simulink model "Set_arm_angles"  (R2020a)
settings: Solver=FixedStepAuto  StartTime=0.0  StopTime=30  FixedStep=0.5  RelTol=1e-3  EnableMultiTasking=on
values from neighbouring files (symbols this model uses):
  initial_elbow_angle = 0*pi/180    (= 0)    [Run_Initializer.m]
  initial_shoulder_angle = 0*pi/180    (= 0)    [Run_Initializer.m]
  initial_wrist_angle = 0*pi/180    (= 0)    [Run_Initializer.m]
settings Model: SimulationMode=external  Creator=AlexC  LastModifiedBy=Kirk
settings SolverCC: PositivePriorityOrder=on
settings DataIOCC: ReturnWorkspaceOutputs=off
settings OptimizationCC: PassReuseOutputArgsThreshold=0  MaxStackSize=64  EfficientTunableParamExpr=on
settings DebuggingCC: ParameterTunabilityLossMsg=error  ArithmeticOperatorsInVariantConditions=warning
settings HardwareCC: ProdBitPerPointer=32  ProdBitPerSizeT=32  ProdBitPerPtrDiffT=32  ProdLargestAtomicInteger=Long  ProdLargestAtomicFloat=Double  ProdWordSize=32  ProdHWDeviceType=ARM Compatible->ARM Cortex
settings SFSimCC: SimUseLocalCustomCode=off  MATLABDynamicMemAlloc=off  CustomCodeUndefinedFunction=UseInterfaceOnly
settings RTWCC: SystemTargetFile=ert.tlc  HardwareBoard=Raspberry Pi  TemplateMakefile=ert_default_tmf  RTWUseLocalCustomCode=off  Toolchain=GNU GCC Raspberry Pi  BuildConfiguration=Specify  TargetLang=C++
settings CodeAppCC: ForceParamTrailComments=on  OperatorAnnotations=on
settings ERTTargetCC: CodeReplacementLibrary=GCC ARM Cortex-A8  ERTCustomFileBanners=off  SupportContinuousTime=on  SupportNonInlinedSFcns=on  RemoveResetFunc=off  SupportVariableSizeSignals=on  ModelStepFunctionPrototypeControlCompliant=off  RootIOFormat=Structure reference

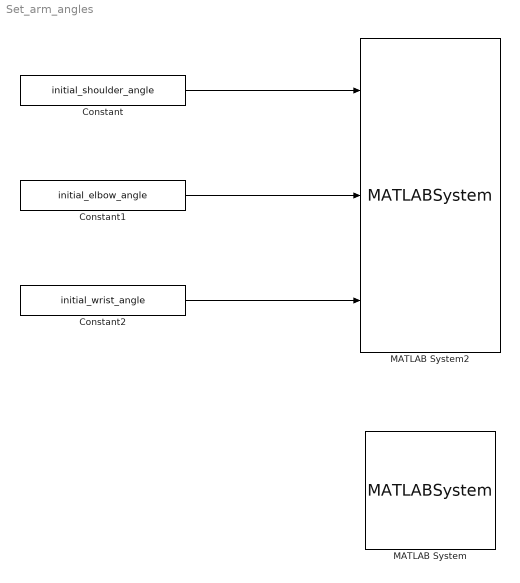
== system Set_arm_angles ==
  Constant : Constant  Value=initial_shoulder_angle
  Constant1 : Constant  Value=initial_elbow_angle
  Constant2 : Constant  Value=initial_wrist_angle
  MATLAB System : MATLABSystem  System=InitializeForPosition  P_GAIN=400  I_GAIN=0  D_GAIN=200  MAX_POSITION=3072  MIN_POSITION=1024  MOVE_TIME=3000
      mask Type: InitializeForPosition
      mask Display: disp('InitializeForPosition');
  MATLAB System2 : MATLABSystem  System=MoveArm_Position
      mask Type: MoveArm_Position
      mask Display:
      | disp('MoveArm_Position');
      | port_label('input',1,'u1');
      | port_label('input',2,'u2');
      | port_label('input',3,'u3');
  wires:
  Constant/1 -> MATLAB System2/1
  Constant2/1 -> MATLAB System2/3
  Constant1/1 -> MATLAB System2/2
